simulink model "Impedance_bis"  (R2020b)
settings: Solver=VariableStepAuto  StartTime=0.0  StopTime=0.5  RelTol=1e-3
values from neighbouring files (symbols this model uses):
  K = diag([3 1 1 2 2 2])    [parameters.m]
  KD = diag([  500   180   160    19     0   8])    [parameters.m]
  KP = diag([2500  3000  1600  100  1  4])    [parameters.m]
  Md = 20*diag([1 1 1 1 1 1])    [parameters.m]
libraries: vrlib x1
settings Model: Creator=Edoardo  LastModifiedBy=Edoardo
settings SolverCC: AlgebraicLoopSolver=LineSearch

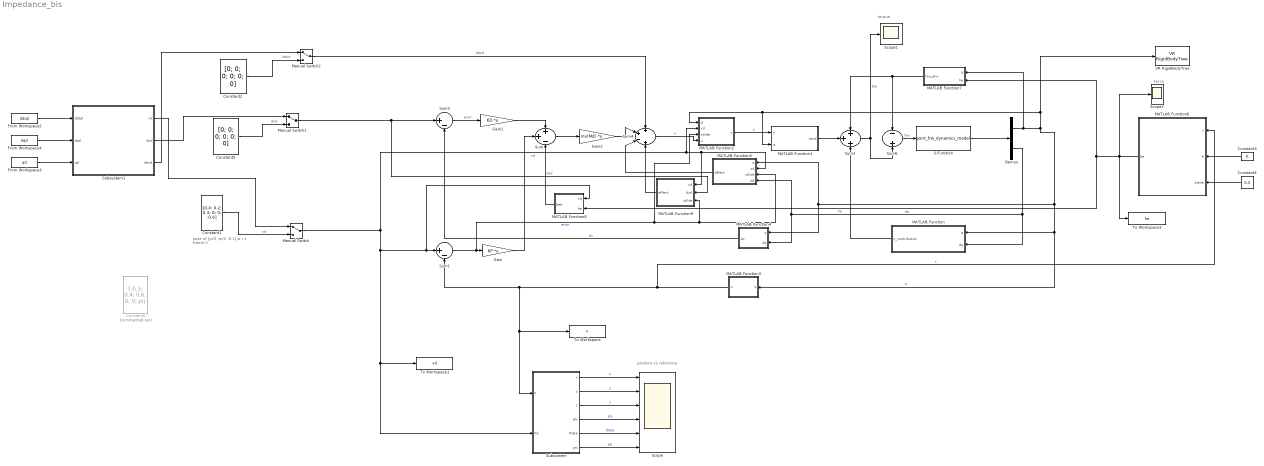
== system Impedance_bis ==
  note: Force
  note: torque
  note: position vs reference
  note: pose of [pi/3 -pi/2 -0.1]
      | w.r.t. frame 0
  Constant1 : Constant  Value=[0.4; 0.2; 0.3; 0; 0; -0.6]  VectorParams1D=off
  Constant2 : Constant  Value=[0; 0; 0; 0; 0; 0]  VectorParams1D=off
  Constant3 : Constant  Value=K
  Constant4 : Constant  Value=0.5
  Constant5 : Constant  Value=[0; 0; 0; 0; 0; 0]  VectorParams1D=off
  Constant6 : Constant  Commented=on  Value=[-0.3; 0.4; 0.6; 0; 0; pi]  VectorParams1D=off
  Demux : Demux  Outputs=2
  From Workspace3 : FromWorkspace  VariableName=qd
  From Workspace4 : FromWorkspace  VariableName=dqd
  From Workspace5 : FromWorkspace  VariableName=ddqd
  Gain : Gain  Gain=KP  Multiplication=Matrix(K*u) (u vector)
  Gain1 : Gain  Gain=KD  Multiplication=Matrix(K*u) (u vector)
  Gain2 : Gain  Gain=inv(Md)  Multiplication=Matrix(K*u) (u vector)
  MATLAB Function : MATLAB Function  TreatAsAtomicUnit=on
  MATLAB Function1 : MATLAB Function  TreatAsAtomicUnit=on
  MATLAB Function2 : MATLAB Function  TreatAsAtomicUnit=on
  MATLAB Function3 : MATLAB Function  TreatAsAtomicUnit=on
  MATLAB Function4 : MATLAB Function  TreatAsAtomicUnit=on
  MATLAB Function5 : MATLAB Function  TreatAsAtomicUnit=on
  MATLAB Function6 : MATLAB Function  TreatAsAtomicUnit=on
  MATLAB Function7 : MATLAB Function  TreatAsAtomicUnit=on
  MATLAB Function8 : MATLAB Function  TreatAsAtomicUnit=on
  MATLAB Function9 : MATLAB Function  TreatAsAtomicUnit=on
  Manual Switch : ManualSwitch
  Manual Switch1 : ManualSwitch
  Manual Switch2 : ManualSwitch
  S-Function : S-Function  FunctionName=joint_frw_dynamics_model  Parameters=myRobot  SFunctionDeploymentMode=off  EnableBusSupport=off
  Scope : Scope  NumInputPorts=6
  Scope1 : Scope
  Scope2 : Scope
  Subsystem : Subsystem
  Subsystem1 : Subsystem
  Sum : Sum  Inputs=++-
  Sum1 : Sum  Inputs=|+-
  Sum2 : Sum  Inputs=|+-
  Sum3 : Sum  Inputs=+++
  Sum4 : Sum  Inputs=++-+
  Sum6 : Sum  Inputs=-+
  To Workspace : ToWorkspace  VariableName=x  SaveFormat=Timeseries  SampleTime=-1
  To Workspace1 : ToWorkspace  VariableName=xd  SaveFormat=Timeseries  SampleTime=-1
  To Workspace2 : ToWorkspace  VariableName=he  SaveFormat=Timeseries  SampleTime=-1
  VR RigidBodyTree : vrlib/VR RigidBodyTree  RBT=robot  useRBT=on  Ts=-1  ForceViewerOpen=on
      settings: SourceProductBaseCode=SL
  wires:
  Sum2/1 -> Gain1/1  "error"
  Sum1/1 -> MATLAB Function9/3(xtilde), MATLAB Function5/3(xtilde), MATLAB Function2/3(xtilde), Gain/1  "error"
  S-Function/1 -> Demux/1
  Sum3/1 -> Sum6/2, Scope1/1  "tau"
  Demux/2 -> MATLAB Function/2(dq), MATLAB Function4/2(dq), MATLAB Function5/4(dq)  "dq"
  Manual Switch1/1 -> Sum2/1, MATLAB Function9/2(dxd)  "dxd"
  Demux/1 -> MATLAB Function7/1(q), MATLAB Function4/1(q), MATLAB Function5/1(q), MATLAB Function3/1(q), MATLAB Function/1(q), VR RigidBodyTree/1, MATLAB Function1/2(q), MATLAB Function2/1(q)  "q"
  MATLAB Function2/1(y) -> MATLAB Function1/1(y)  "y"
  MATLAB Function4/1(dx) -> Sum2/2  "dx"
  Subsystem/1(x) -> Scope/1  "x"
  Subsystem/4(phi) -> Scope/4  "phi"
  Subsystem/6(psi) -> Scope/6  "psi"
  Subsystem/2(y) -> Scope/2  "y"
  Subsystem/5(theta) -> Scope/5  "theta"
  MATLAB Function3/1(x) -> MATLAB Function6/1(x), To Workspace/1, Subsystem/1(X), Sum1/2  "x"
  Manual Switch/1 -> MATLAB Function9/1(xd), MATLAB Function5/2(xd), MATLAB Function2/2(xd), Sum1/1, MATLAB Function8/1(xd), To Workspace1/1, Subsystem/2(Xd)  "xd"
  Subsystem/3(z) -> Scope/3  "z"
  Constant4/1 -> MATLAB Function6/3(plane)
  Constant3/1 -> MATLAB Function6/2(K)
  MATLAB Function6/1(he) -> To Workspace2/1, MATLAB Function7/2(he), MATLAB Function8/2(he), Scope2/1  "he"
  MATLAB Function/1(n_contribution) -> Sum3/3
  MATLAB Function1/1(taud) -> Sum3/2
  MATLAB Function7/1(tau_env) -> Sum6/1, Sum3/1
  Sum4/1 -> MATLAB Function2/4(u)  "u"
  MATLAB Function5/1(effect) -> Sum4/3
  MATLAB Function8/1(hed) -> Sum/3
  Gain1/1 -> Sum/1
  Gain/1 -> Sum/2
  Manual Switch2/1 -> Sum4/1  "ddxd"
  Gain2/1 -> Sum4/2
  Sum/1 -> Gain2/1
  Sum6/1 -> S-Function/1  "tau"
  Subsystem1/1(xd) -> Manual Switch/1
  Constant1/1 -> Manual Switch/2  "xd"
  Constant5/1 -> Manual Switch1/2  "dxd"
  Subsystem1/2(dxd) -> Manual Switch1/1
  Constant2/1 -> Manual Switch2/2  "ddxd"
  Subsystem1/3(ddxd) -> Manual Switch2/1
  From Workspace4/1 -> Subsystem1/2(dqd)
  From Workspace3/1 -> Subsystem1/3(qd)
  From Workspace5/1 -> Subsystem1/1(ddqd)
  MATLAB Function9/1(effect) -> Sum4/4

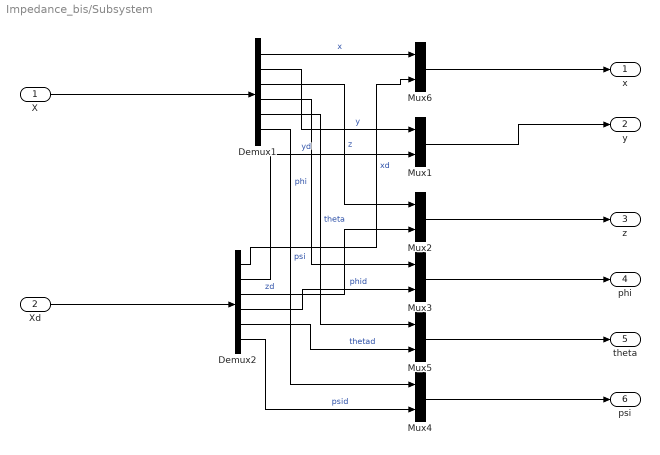
== system Impedance_bis/Subsystem ==
  X : Inport
  Xd : Inport  Port=2
  Demux1 : Demux  Outputs=6
  Demux2 : Demux  Outputs=6
  Mux{1..6} (6 alike) : Mux  Inputs=2
  x : Outport
  y : Outport  Port=2
  z : Outport  Port=3
  phi : Outport  Port=4
  theta : Outport  Port=5
  psi : Outport  Port=6
  wires:
  Demux1/3 -> Mux2/1  "z"
  Demux1/4 -> Mux3/1  "phi"
  Demux2/3 -> Mux2/2  "zd"
  Mux2/1 -> z/1
  Demux2/1 -> Mux6/2  "xd"
  Demux1/5 -> Mux5/1  "theta"
  Mux1/1 -> y/1
  Demux1/6 -> Mux4/1  "psi"
  Demux1/1 -> Mux6/1  "x"
  Demux2/5 -> Mux5/2  "thetad"
  Demux2/6 -> Mux4/2  "psid"
  Demux1/2 -> Mux1/1  "y"
  Demux2/4 -> Mux3/2  "phid"
  Demux2/2 -> Mux1/2  "yd"
  Xd/1 -> Demux2/1
  X/1 -> Demux1/1
  Mux3/1 -> phi/1
  Mux5/1 -> theta/1
  Mux4/1 -> psi/1
  Mux6/1 -> x/1

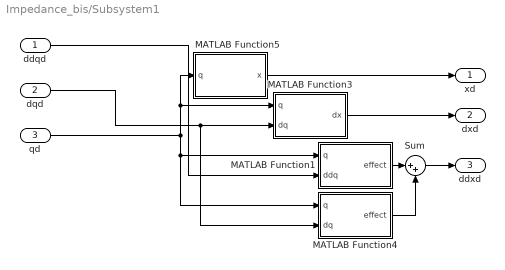
== system Impedance_bis/Subsystem1 ==
  ddqd : Inport
  dqd : Inport  Port=2
  qd : Inport  Port=3
  MATLAB Function1 : MATLAB Function  TreatAsAtomicUnit=on
  MATLAB Function3 : MATLAB Function  TreatAsAtomicUnit=on
  MATLAB Function4 : MATLAB Function  TreatAsAtomicUnit=on
  MATLAB Function5 : MATLAB Function  TreatAsAtomicUnit=on
  Sum : Sum  Inputs=|++
  xd : Outport
  dxd : Outport  Port=2
  ddxd : Outport  Port=3
  wires:
  Sum/1 -> ddxd/1
  qd/1 -> MATLAB Function5/1(q), MATLAB Function3/1(q), MATLAB Function4/1(q), MATLAB Function1/1(q)
  MATLAB Function4/1(effect) -> Sum/2
  MATLAB Function3/1(dx) -> dxd/1
  dqd/1 -> MATLAB Function3/2(dq), MATLAB Function4/2(dq)
  MATLAB Function1/1(effect) -> Sum/1
  ddqd/1 -> MATLAB Function1/2(ddq)
  MATLAB Function5/1(x) -> xd/1

== matlab function Impedance_bis/Subsystem1/MATLAB Function1 ==
  data: q input; effect output; ddq input
function effect = JA(q, ddq)

effect = getAnalyticalJacobian(q)*ddq;

== matlab function Impedance_bis/Subsystem1/MATLAB Function4 ==
  data: q input; effect output; dq input
function effect = dJA(q, dq)


effect = getDAnalyticalJacobian(q, dq)*dq;

== matlab function Impedance_bis/Subsystem1/MATLAB Function5 ==
  data: q input; x output
function x = K(q)

t1 = q(1);
t2 = q(2);
d3 = q(3);

K = [[ cos(t1 + t2), -sin(t1 + t2), 0, (3*cos(t1 + t2))/10 + (2*cos(t1))/5]
     [ sin(t1 + t2),  cos(t1 + t2), 0, (3*sin(t1 + t2))/10 + (2*sin(t1))/5]
     [            0,             0, 1,                            d3 + 2/5]
     [            0,             0, 0,                                   1]];

pos = K(1:3, 4);
ori = rotm2eul(K(1:3,1:3), 'ZYZ')';

x = [pos; ori];

== matlab function Impedance_bis/MATLAB Function9 ==
  data: xd input; dxd input; effect output; xtilde input
function effect = db(xd, dxd, xtilde)

R = eul2rotm(xd(4:6)', 'ZYZ');

do = dxd(1:3);
wd = dxd(4:6);

o = xd(1:3);

[Ta, Tphi] = getTransformAnalytical(xtilde(4:6));
Tinv = pinv(Tphi);

wx = wd(1);
wy = wd(2);
wz = wd(3);
S = [0 -wz wy 
     wz 0 -wx 
     -wy wx 0 ];
 
effect = [R'*do + S*o; 
            Tinv*wd   ];

== matlab function Impedance_bis/MATLAB Function1 ==
  data: y input; taud output; q input size=3
function taud = B(y, q)

    taud = getBHatLagrangian(q)*y;

== matlab function Impedance_bis/MATLAB Function ==
  data: q input size=3; n_contribution output; dq input size=3
function n_contribution = n(q,dq)
    n_contribution = getCHatLagrangian(q,dq)*dq + getGHatLagrangian(q);

== matlab function Impedance_bis/MATLAB Function2 ==
  data: q input; xd input; xtilde input; u input; y output
function y = JAd_inv(q,xd, xtilde, u)

% Compute the rotational matrix of the desired fame xd
R = eul2rotm(xd(4:6)', 'ZYZ');

% Compute the analytical jacobian respect to the desired frame 
Jad = pinv(getTransformAnalytical(xtilde(4:6)))*[R', zeros(3,3); zeros(3,3), R']*getJacobian(q);

y = pinv(Jad)*u;

== matlab function Impedance_bis/MATLAB Function3 ==
  data: q input size=3; x output size=6
function x = K(q)

K = getDirectKinematics(q);

pos = K(1:3, 4);
rotm = K(1:3,1:3); 
ori = rotm2eul(rotm, 'ZYZ')';

x = [pos; ori];

== matlab function Impedance_bis/MATLAB Function4 ==
  data: q input size=3; dx output size=6; dq input size=3
function dx = JA(q,dq)

dx = getAnalyticalJacobian(q)*dq;

== matlab function Impedance_bis/MATLAB Function5 ==
  data: q input; xd input; xtilde input; effect output; dq input
function effect = dJAd(q, xd, xtilde, dq)

    
% Compute the rotational matrix of the desired fame xd
R = eul2rotm(xd(4:6)', 'ZYZ');

% Compute the analytical jacobian respect to the desired frame 
Jad = pinv(getTransformAnalytical(xtilde(4:6)))*[R', zeros(3,3); zeros(3,3), R']*getJacobian(q);
%dJad = computeDAnalyticalJacobian(Jad, q, dq);

effect = Jad*dq;

== matlab function Impedance_bis/MATLAB Function6 ==
  data: x input; he output; K input; plane input
function he = environment(x, K, plane)

% The robot is touching the environment! constrained motion
if x(2) >= plane
   
    xr = zeros(6,1);
    xr(2) = plane;
    
    % compute the forces 
    xe = zeros(6,1);
    xe(2) = x(2);

    he = K * (xe - xr);

% free motion
else
    
    he = zeros(6,1);
    
end

== matlab function Impedance_bis/MATLAB Function7 ==
  data: q input; he input; tau_env output
function tau_env = JT(q, he)

tau_env = getJacobian(q)'*he;

== matlab function Impedance_bis/Subsystem1/MATLAB Function3 ==
  data: q input; dx output; dq input
function dx = JA(q, dq)

dx = getAnalyticalJacobian(q)*dq;

== matlab function Impedance_bis/MATLAB Function8 ==
  data: xd input; hed output; he input
function hed = TAT(xd,he)

orientation = xd(4:6);
hed = getTransformAnalytical(orientation)'*he;
